simulink library "ssc_Probes_2014a"  (R2019b)
settings: Solver=ode45  StartTime=0.0  StopTime=10.0  RelTol=1e-3  EnableMultiTasking=on
libraries: fl_lib x50, nesl_utility x49, pe_lib x9
(part 3 of 3)

== system ssc_Probes_2014a/Pneumatic/AbsTemperature ==
  PS-S : nesl_utility/PS-Simulink Converter  PhysicalDomain=network_engine_domain  SubClassName=ps_output  LeftPortType=input  RightPortType=output  PseudoPeriodic=off  Frequencies=[]  Unit=K  AffineConversion=off
  Pneumatic Absolute Reference : fl_lib/Pneumatic/Pneumatic Elements/Pneumatic Absolute Reference  G_Log=off  Q_Log=off  LocalVarNames=|G|Q  LocalVarDescs=|G|Q  LocalVarLogging=[0 0]
      settings: SourceProductName=Simscape  SourceProductBaseCode=SS
  Pneumatic Pressure & Temperature Sensor : fl_lib/Pneumatic/Pneumatic Sensors/Pneumatic Pressure & Temperature Sensor
      settings: SourceProductName=Simscape  SourceProductBaseCode=SS
  Terminator : Terminator
  A : PMIOPort  Side=Left
  wires:
  PS-S/1 -> [AbsTemperature]  "AbsTemperature"
  [AbsTemperature] -> Terminator/1
  connections:
  PS-S/LConn1 -- Pneumatic Pressure & Temperature Sensor/RConn3
  Pneumatic Absolute Reference/LConn1 -- Pneumatic Pressure & Temperature Sensor/RConn1
  A/RConn1 -- Pneumatic Pressure & Temperature Sensor/LConn1

== system ssc_Probes_2014a/Pneumatic/AtmTemperature ==
  PS-S : nesl_utility/PS-Simulink Converter  PhysicalDomain=network_engine_domain  SubClassName=ps_output  LeftPortType=input  RightPortType=output  PseudoPeriodic=off  Frequencies=[]  Unit=K  AffineConversion=off
  Pneumatic Atmospheric Reference : fl_lib/Pneumatic/Pneumatic Elements/Pneumatic Atmospheric Reference  gas_flow_Log=off  heat_flow_Log=off  LocalVarNames=|gas_flow|heat_flow  LocalVarDescs=|gas_flow|heat_flow  LocalVarLogging=[0 0]
      settings: SourceProductName=Simscape  SourceProductBaseCode=SS
  Pneumatic Pressure & Temperature Sensor : fl_lib/Pneumatic/Pneumatic Sensors/Pneumatic Pressure & Temperature Sensor
      settings: SourceProductName=Simscape  SourceProductBaseCode=SS
  Terminator : Terminator
  A : PMIOPort  Side=Left
  wires:
  PS-S/1 -> [AtmTemperature]  "AtmTemperature"
  [AtmTemperature] -> Terminator/1
  connections:
  A/RConn1 -- Pneumatic Pressure & Temperature Sensor/LConn1
  Pneumatic Atmospheric Reference/LConn1 -- Pneumatic Pressure & Temperature Sensor/RConn1
  PS-S/LConn1 -- Pneumatic Pressure & Temperature Sensor/RConn3

== system ssc_Probes_2014a/Pneumatic/GasHeatFlow ==
  PS-S : nesl_utility/PS-Simulink Converter  PhysicalDomain=network_engine_domain  SubClassName=ps_output  LeftPortType=input  RightPortType=output  PseudoPeriodic=off  Frequencies=[]  Unit=J/s  AffineConversion=off
  Pneumatic Mass & Heat Flow Sensor : fl_lib/Pneumatic/Pneumatic Sensors/Pneumatic Mass & Heat Flow Sensor
      settings: SourceProductName=Simscape  SourceProductBaseCode=SS
  Terminator : Terminator
  A : PMIOPort  Side=Left
  B : PMIOPort  Port=2  Side=Right
  wires:
  PS-S/1 -> [GasHeatFlow]  "GasHeatFlow"
  [GasHeatFlow] -> Terminator/1
  connections:
  PS-S/LConn1 -- Pneumatic Mass & Heat Flow Sensor/RConn3
  B/RConn1 -- Pneumatic Mass & Heat Flow Sensor/RConn1
  A/RConn1 -- Pneumatic Mass & Heat Flow Sensor/LConn1

== system ssc_Probes_2014a/Pneumatic/GaugePressure ==
  PS-S : nesl_utility/PS-Simulink Converter  PhysicalDomain=network_engine_domain  SubClassName=ps_output  LeftPortType=input  RightPortType=output  PseudoPeriodic=off  Frequencies=[]  Unit=Pa  AffineConversion=off
  Pneumatic Atmospheric Reference : fl_lib/Pneumatic/Pneumatic Elements/Pneumatic Atmospheric Reference  gas_flow_Log=off  heat_flow_Log=off  LocalVarNames=|gas_flow|heat_flow  LocalVarDescs=|gas_flow|heat_flow  LocalVarLogging=[0 0]
      settings: SourceProductName=Simscape  SourceProductBaseCode=SS
  Pneumatic Pressure & Temperature Sensor : fl_lib/Pneumatic/Pneumatic Sensors/Pneumatic Pressure & Temperature Sensor
      settings: SourceProductName=Simscape  SourceProductBaseCode=SS
  Terminator : Terminator
  A : PMIOPort  Side=Left
  wires:
  PS-S/1 -> [GaugePressure]  "GaugePressure"
  [GaugePressure] -> Terminator/1
  connections:
  PS-S/LConn1 -- Pneumatic Pressure & Temperature Sensor/RConn2
  Pneumatic Atmospheric Reference/LConn1 -- Pneumatic Pressure & Temperature Sensor/RConn1
  A/RConn1 -- Pneumatic Pressure & Temperature Sensor/LConn1

== system ssc_Probes_2014a/Pneumatic/MassFlow ==
  PS-S : nesl_utility/PS-Simulink Converter  PhysicalDomain=network_engine_domain  SubClassName=ps_output  LeftPortType=input  RightPortType=output  PseudoPeriodic=off  Frequencies=[]  Unit=kg/s  AffineConversion=off
  Pneumatic Mass & Heat Flow Sensor : fl_lib/Pneumatic/Pneumatic Sensors/Pneumatic Mass & Heat Flow Sensor
      settings: SourceProductName=Simscape  SourceProductBaseCode=SS
  Terminator : Terminator
  A : PMIOPort  Side=Left
  B : PMIOPort  Port=2  Side=Right
  wires:
  PS-S/1 -> [MassFlow]  "MassFlow"
  [MassFlow] -> Terminator/1
  connections:
  A/RConn1 -- Pneumatic Mass & Heat Flow Sensor/LConn1
  Pneumatic Mass & Heat Flow Sensor/RConn2 -- PS-S/LConn1
  B/RConn1 -- Pneumatic Mass & Heat Flow Sensor/RConn1

== system ssc_Probes_2014a/Pneumatic/dGasPressure ==
  PS-S : nesl_utility/PS-Simulink Converter  PhysicalDomain=network_engine_domain  SubClassName=ps_output  LeftPortType=input  RightPortType=output  PseudoPeriodic=off  Frequencies=[]  Unit=Pa  AffineConversion=off
  Pneumatic Pressure & Temperature Sensor : fl_lib/Pneumatic/Pneumatic Sensors/Pneumatic Pressure & Temperature Sensor
      settings: SourceProductName=Simscape  SourceProductBaseCode=SS
  Terminator : Terminator
  A : PMIOPort  Side=Left
  B : PMIOPort  Port=2  Side=Right
  wires:
  PS-S/1 -> [dGasPressure]  "dGasPressure"
  [dGasPressure] -> Terminator/1
  connections:
  A/RConn1 -- Pneumatic Pressure & Temperature Sensor/LConn1
  B/RConn1 -- Pneumatic Pressure & Temperature Sensor/RConn1
  Pneumatic Pressure & Temperature Sensor/RConn2 -- PS-S/LConn1

== system ssc_Probes_2014a/Pneumatic/dGasTemperature ==
  PS-S : nesl_utility/PS-Simulink Converter  PhysicalDomain=network_engine_domain  SubClassName=ps_output  LeftPortType=input  RightPortType=output  PseudoPeriodic=off  Frequencies=[]  Unit=K  AffineConversion=off
  Pneumatic Pressure & Temperature Sensor : fl_lib/Pneumatic/Pneumatic Sensors/Pneumatic Pressure & Temperature Sensor
      settings: SourceProductName=Simscape  SourceProductBaseCode=SS
  Terminator : Terminator
  A : PMIOPort  Side=Left
  B : PMIOPort  Port=2  Side=Right
  wires:
  PS-S/1 -> [dGasTemperature]  "dGasTemperature"
  [dGasTemperature] -> Terminator/1
  connections:
  PS-S/LConn1 -- Pneumatic Pressure & Temperature Sensor/RConn3
  B/RConn1 -- Pneumatic Pressure & Temperature Sensor/RConn1
  A/RConn1 -- Pneumatic Pressure & Temperature Sensor/LConn1

== system ssc_Probes_2014a/Thermal/HeatFlow ==
  Ideal Heat Flow Sensor : fl_lib/Thermal/Thermal Sensors/Ideal Heat Flow Sensor
      settings: SourceProductName=Simscape  SourceProductBaseCode=SS
  PS-S : nesl_utility/PS-Simulink Converter  PhysicalDomain=network_engine_domain  SubClassName=ps_output  LeftPortType=input  RightPortType=output  PseudoPeriodic=off  Frequencies=[]  Unit=J/s  AffineConversion=off
  Terminator : Terminator
  A : PMIOPort  Side=Left
  B : PMIOPort  Port=2  Side=Right
  wires:
  PS-S/1 -> [HeatFlow]  "HeatFlow"
  [HeatFlow] -> Terminator/1
  connections:
  A/RConn1 -- Ideal Heat Flow Sensor/LConn1
  Ideal Heat Flow Sensor/RConn1 -- PS-S/LConn1
  B/RConn1 -- Ideal Heat Flow Sensor/RConn2

== system ssc_Probes_2014a/Thermal/Temperature ==
  Ideal Temperature Sensor : fl_lib/Thermal/Thermal Sensors/Ideal Temperature Sensor
      settings: SourceProductName=Simscape  SourceProductBaseCode=SS
  PS-S : nesl_utility/PS-Simulink Converter  PhysicalDomain=network_engine_domain  SubClassName=ps_output  LeftPortType=input  RightPortType=output  PseudoPeriodic=off  Frequencies=[]  Unit=K  AffineConversion=off
  Terminator : Terminator
  Thermal Reference : fl_lib/Thermal/Thermal Elements/Thermal Reference  Q_Log=off  LocalVarNames=|Q  LocalVarDescs=|Q  LocalVarLogging=0
  A : PMIOPort  Side=Left
  wires:
  PS-S/1 -> [Temperature]  "Temperature"
  [Temperature] -> Terminator/1
  connections:
  A/RConn1 -- Ideal Temperature Sensor/LConn1
  Thermal Reference/LConn1 -- Ideal Temperature Sensor/RConn1
  PS-S/LConn1 -- Ideal Temperature Sensor/RConn2

== system ssc_Probes_2014a/Thermal/dTemperature ==
  Ideal Temperature Sensor : fl_lib/Thermal/Thermal Sensors/Ideal Temperature Sensor
      settings: SourceProductName=Simscape  SourceProductBaseCode=SS
  PS-S : nesl_utility/PS-Simulink Converter  PhysicalDomain=network_engine_domain  SubClassName=ps_output  LeftPortType=input  RightPortType=output  PseudoPeriodic=off  Frequencies=[]  Unit=K  AffineConversion=off
  Terminator : Terminator
  A : PMIOPort  Side=Left
  B : PMIOPort  Port=2  Side=Right
  wires:
  PS-S/1 -> [dTemperature]  "dTemperature"
  [dTemperature] -> Terminator/1
  connections:
  PS-S/LConn1 -- Ideal Temperature Sensor/RConn2
  B/RConn1 -- Ideal Temperature Sensor/RConn1
  A/RConn1 -- Ideal Temperature Sensor/LConn1

== system ssc_Probes_2014a/ThermalLiquid/AbsPressure_TL ==
  Absolute Reference (TL) : fl_lib/Thermal Liquid/Elements/Absolute Reference (TL)  mdot_Log=off  Phi_Log=off  LocalVarNames=|mdot|Phi  LocalVarDescs=|mdot|Phi  LocalVarLogging=[0 0]
      settings: SourceProductName=Simscape  SourceProductBaseCode=SS
  PS-S : nesl_utility/PS-Simulink Converter  PhysicalDomain=network_engine_domain  SubClassName=ps_output  LeftPortType=input  RightPortType=output  PseudoPeriodic=off  Frequencies=[]  Unit=Pa  AffineConversion=off
  Pressure & Temperature Sensor (TL) : fl_lib/Thermal Liquid/Sensors/Pressure & Temperature Sensor (TL)
      settings: SourceProductName=Simscape  SourceProductBaseCode=SS
  Terminator : Terminator
  A : PMIOPort  Side=Left
  wires:
  PS-S/1 -> [AbsPressure_TL]  "AbsPressure_TL"
  [AbsPressure_TL] -> Terminator/1
  connections:
  Absolute Reference (TL)/LConn1 -- Pressure & Temperature Sensor (TL)/RConn1
  Pressure & Temperature Sensor (TL)/LConn1 -- A/RConn1
  PS-S/LConn1 -- Pressure & Temperature Sensor (TL)/RConn2

== system ssc_Probes_2014a/ThermalLiquid/AbsTemperature_TL ==
  Absolute Reference (TL) : fl_lib/Thermal Liquid/Elements/Absolute Reference (TL)  mdot_Log=off  Phi_Log=off  LocalVarNames=|mdot|Phi  LocalVarDescs=|mdot|Phi  LocalVarLogging=[0 0]
      settings: SourceProductName=Simscape  SourceProductBaseCode=SS
  PS-S : nesl_utility/PS-Simulink Converter  PhysicalDomain=network_engine_domain  SubClassName=ps_output  LeftPortType=input  RightPortType=output  PseudoPeriodic=off  Frequencies=[]  Unit=K  AffineConversion=off
  Pressure & Temperature Sensor (TL) : fl_lib/Thermal Liquid/Sensors/Pressure & Temperature Sensor (TL)
      settings: SourceProductName=Simscape  SourceProductBaseCode=SS
  Terminator : Terminator
  A : PMIOPort  Side=Left
  wires:
  [AbsTemperature_TL] -> Terminator/1
  PS-S/1 -> [AbsTemperature_TL]  "AbsTemperature_TL"
  connections:
  PS-S/LConn1 -- Pressure & Temperature Sensor (TL)/RConn3
  Pressure & Temperature Sensor (TL)/LConn1 -- A/RConn1
  Absolute Reference (TL)/LConn1 -- Pressure & Temperature Sensor (TL)/RConn1

== system ssc_Probes_2014a/ThermalLiquid/MassFlow_TL ==
  Mass Flow Rate & Thermal Flux Sensor (TL) : fl_lib/Thermal Liquid/Sensors/Mass Flow Rate & Thermal Flux Sensor (TL)
      settings: SourceProductName=Simscape  SourceProductBaseCode=SS
  PS-S : nesl_utility/PS-Simulink Converter  PhysicalDomain=network_engine_domain  SubClassName=ps_output  LeftPortType=input  RightPortType=output  PseudoPeriodic=off  Frequencies=[]  Unit=kg/s  AffineConversion=off
  Terminator : Terminator
  A : PMIOPort  Side=Left
  B : PMIOPort  Port=2  Side=Right
  wires:
  [MassFlow_TL] -> Terminator/1
  PS-S/1 -> [MassFlow_TL]  "MassFlow_TL"
  connections:
  Mass Flow Rate & Thermal Flux Sensor (TL)/RConn1 -- B/RConn1
  PS-S/LConn1 -- Mass Flow Rate & Thermal Flux Sensor (TL)/RConn2
  Mass Flow Rate & Thermal Flux Sensor (TL)/LConn1 -- A/RConn1

== system ssc_Probes_2014a/ThermalLiquid/ThermalFlux_TL ==
  Mass Flow Rate & Thermal Flux Sensor (TL) : fl_lib/Thermal Liquid/Sensors/Mass Flow Rate & Thermal Flux Sensor (TL)
      settings: SourceProductName=Simscape  SourceProductBaseCode=SS
  PS-S : nesl_utility/PS-Simulink Converter  PhysicalDomain=network_engine_domain  SubClassName=ps_output  LeftPortType=input  RightPortType=output  PseudoPeriodic=off  Frequencies=[]  Unit=J/s  AffineConversion=off
  Terminator : Terminator
  A : PMIOPort  Side=Left
  B : PMIOPort  Port=2  Side=Right
  wires:
  PS-S/1 -> [ThermalFlux_TL]  "ThermalFlux_TL"
  [ThermalFlux_TL] -> Terminator/1
  connections:
  Mass Flow Rate & Thermal Flux Sensor (TL)/LConn1 -- A/RConn1
  Mass Flow Rate & Thermal Flux Sensor (TL)/RConn1 -- B/RConn1
  Mass Flow Rate & Thermal Flux Sensor (TL)/RConn3 -- PS-S/LConn1

== system ssc_Probes_2014a/ThermalLiquid/dPressure_TL ==
  PS-S : nesl_utility/PS-Simulink Converter  PhysicalDomain=network_engine_domain  SubClassName=ps_output  LeftPortType=input  RightPortType=output  PseudoPeriodic=off  Frequencies=[]  Unit=Pa  AffineConversion=off
  Pressure & Temperature Sensor (TL) : fl_lib/Thermal Liquid/Sensors/Pressure & Temperature Sensor (TL)
      settings: SourceProductName=Simscape  SourceProductBaseCode=SS
  Terminator : Terminator
  A : PMIOPort  Side=Left
  B : PMIOPort  Port=2  Side=Right
  wires:
  PS-S/1 -> [dPressure_TL]  "dPressure_TL"
  [dPressure_TL] -> Terminator/1
  connections:
  B/RConn1 -- Pressure & Temperature Sensor (TL)/RConn1
  Pressure & Temperature Sensor (TL)/LConn1 -- A/RConn1
  Pressure & Temperature Sensor (TL)/RConn2 -- PS-S/LConn1

== system ssc_Probes_2014a/ThermalLiquid/dTemperature_TL ==
  PS-S : nesl_utility/PS-Simulink Converter  PhysicalDomain=network_engine_domain  SubClassName=ps_output  LeftPortType=input  RightPortType=output  PseudoPeriodic=off  Frequencies=[]  Unit=K  AffineConversion=off
  Pressure & Temperature Sensor (TL) : fl_lib/Thermal Liquid/Sensors/Pressure & Temperature Sensor (TL)
      settings: SourceProductName=Simscape  SourceProductBaseCode=SS
  Terminator : Terminator
  A : PMIOPort  Side=Left
  B : PMIOPort  Port=2  Side=Right
  wires:
  [dTemperature_TL] -> Terminator/1
  PS-S/1 -> [dTemperature_TL]  "dTemperature_TL"
  connections:
  Pressure & Temperature Sensor (TL)/LConn1 -- A/RConn1
  B/RConn1 -- Pressure & Temperature Sensor (TL)/RConn1
  PS-S/LConn1 -- Pressure & Temperature Sensor (TL)/RConn3
